simulink model "EX1_B"  (R2017b)
settings: Solver=VariableStepAuto  StartTime=0.0  StopTime=10.0  RelTol=1e-3
settings Model: Creator=yanub  LastModifiedBy=yanub

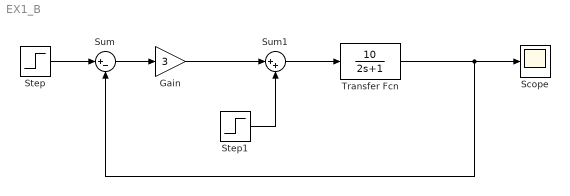
== system EX1_B ==
  Gain : Gain  Gain=3
  Scope : Scope
  Step : Step  SampleTime=0
  Step1 : Step  SampleTime=0
  Sum : Sum  Inputs=|+-
  Sum1 : Sum  Inputs=|++
  Transfer Fcn : TransferFcn  Numerator=[10]  Denominator=[2 1]
  wires:
  Transfer Fcn/1 -> Sum/2, Scope/1
  Step1/1 -> Sum1/2
  Sum1/1 -> Transfer Fcn/1
  Gain/1 -> Sum1/1
  Step/1 -> Sum/1
  Sum/1 -> Gain/1
